simulink model "Capitulo12pg432"  (R2020a)
settings: Solver=VariableStepAuto  StartTime=0.0  StopTime=10  MaxStep=1e-3  RelTol=1e-3
undefined symbols (not defined in the file): d, n, wn, zeta
settings Model: Creator=a1  LastModifiedBy=a1

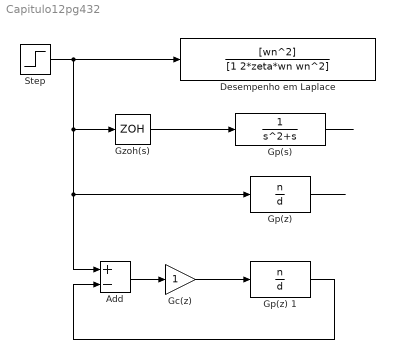
== system Capitulo12pg432 ==
  " Desempenho em Laplace" : TransferFcn  Numerator=[wn^2]  Denominator=[1 2*zeta*wn wn^2]
  Add : Sum  Inputs=+-
  Gc(z) : Gain
  "Gp(s) " : TransferFcn  Denominator=[1 1 0]
  "Gp(z) " : DiscreteTransferFcn  Numerator=n  Denominator=d  SampleTime=0.2
  Gp(z) 1 : DiscreteTransferFcn  Numerator=n  Denominator=d  SampleTime=0.2
  Gzoh(s) : ZeroOrderHold  SampleTime=0.2
  Step : Step  SampleTime=0
  wires:
  Step/1 -> Add/1, "Gp(z) "/1, Gzoh(s)/1, " Desempenho em Laplace"/1
  Gzoh(s)/1 -> "Gp(s) "/1
  "Gp(s) "/1 -> ?
  "Gp(z) "/1 -> ?
  Add/1 -> Gc(z)/1
  Gc(z)/1 -> Gp(z) 1/1
  Gp(z) 1/1 -> Add/2
